simulink model "simulink1"  (R2014a)
settings: Solver=FixedStepDiscrete  StartTime=0.0  StopTime=20.0  FixedStep=0.01  RelTol=1e-3
settings Model: Creator=Abhay  LastModifiedBy=Abhay

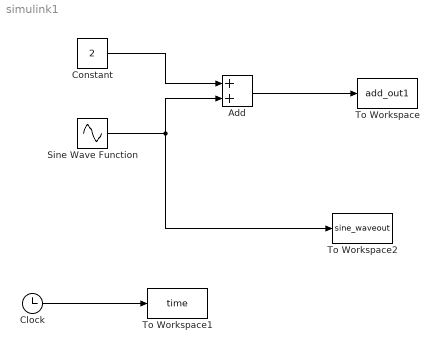
== system simulink1 ==
  Add : Sum
  Clock : Clock
  Constant : Constant  Value=2
  Sine Wave Function : Sin  Amplitude=5  SampleTime=0
  To Workspace : ToWorkspace  VariableName=add_out1  SampleTime=-1
  To Workspace1 : ToWorkspace  VariableName=time  SampleTime=-1
  To Workspace2 : ToWorkspace  VariableName=sine_waveout  SampleTime=-1
  wires:
  Constant/1 -> Add/1
  Sine Wave Function/1 -> To Workspace2/1, Add/2
  Add/1 -> To Workspace/1
  Clock/1 -> To Workspace1/1
